simulink model "PIL_controller"  (R2022b)
settings: Solver=FixedStepAuto  StartTime=0.0  StopTime=10.0  FixedStep=0.01  RelTol=1e-3  EnableMultiTasking=on
libraries: pil_lib x1
settings Model: Creator=ok  LastModifiedBy=ok
settings OptimizationCC: EnhancedBackFolding=on  PassReuseOutputArgsAs=Individual arguments  ZeroExternalMemoryAtStartup=off  ZeroInternalMemoryAtStartup=off  MaxStackSize=64  OptimizeBlockOrder=speed  DifferentSizesBufferReuse=on  OptimizationCustomize=off  EfficientTunableParamExpr=on
settings DebuggingCC: ParameterTunabilityLossMsg=error
settings HardwareCC: ProdBitPerInt=16  ProdBitPerPointer=16  ProdBitPerSizeT=16  ProdBitPerPtrDiffT=16  ProdLargestAtomicFloat=None  ProdWordSize=8  ProdHWDeviceType=Atmel->AVR
settings SFSimCC: MATLABDynamicMemAlloc=off
settings RTWCC: Description=Embedded Coder  SystemTargetFile=ert.tlc  HardwareBoard=Arduino Uno  TLCOptions=-aInlineSetEventsForThisBaseRateFcn=TLC_FALSE -aSuppressMultiTaskScheduler=TLC_FALSE -aRateBasedStepFcn=1  TemplateMakefile=ert_default_tmf  Toolchain=Arduino AVR  BuildConfiguration=Faster Runs  CreateSILPILBlock=PIL
settings CodeAppCC: ForceParamTrailComments=on  IgnoreCustomStorageClasses=off  OperatorAnnotations=on  SimulinkDataObjDesc=on  SFDataObjDesc=on  InsertBlockDesc=on
settings ERTTargetCC: SupportContinuousTime=on  SupportVariableSizeSignals=on  ExtModeTransport=3  ExtModeStaticAlloc=on  ExtModeAutomaticAllocSize=off  ExtModeStaticAllocSize=250  ExtModeMexFile=ext_xcp  ExtModeIntrfLevel=Level2 - Open

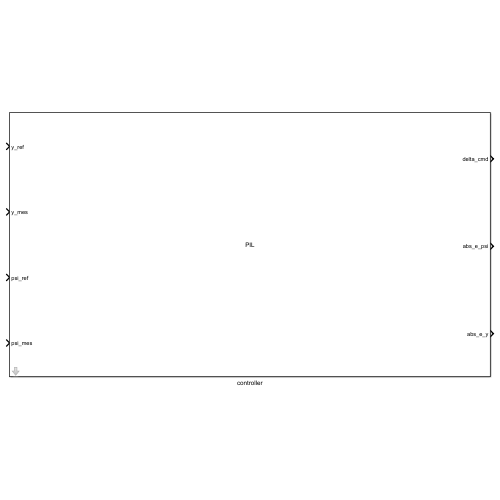
[thumbnail: Simulink's stored preview of the top-level diagram]
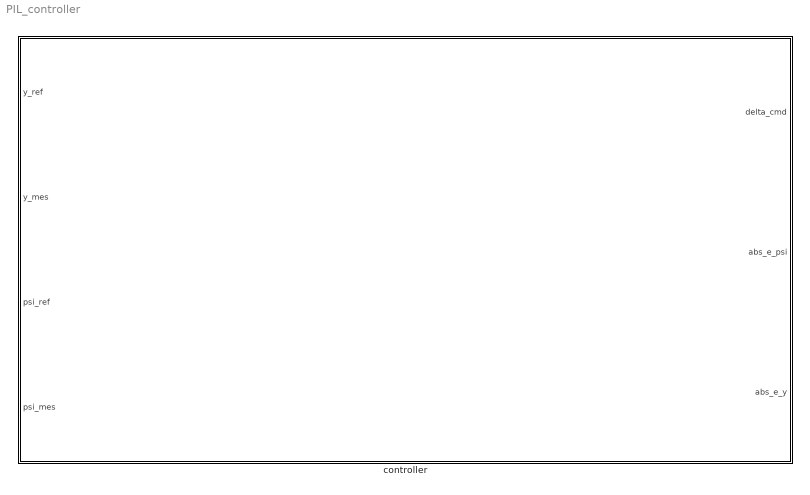
== system PIL_controller ==
  controller : Subsystem  DialogController=pil_create_dialog  LoadFcn=|
      | try
      |    if ~strcmp(rtw.pil.getPILVersion, '9.13 (R2022b)_15')
      |       set_param(gcb, 'DialogController', '');
      |       set_param(gcb, 'DialogControllerArgs', '');
      |    end
      | catch e
      |       set_param(gcb, 'DialogController', '');
      |       set_param(gcb, 'DialogControllerArgs', '');
      | end
      mask help: PIL:pil:XILBlockMaskDesc
      mask Display: disp('PIL');

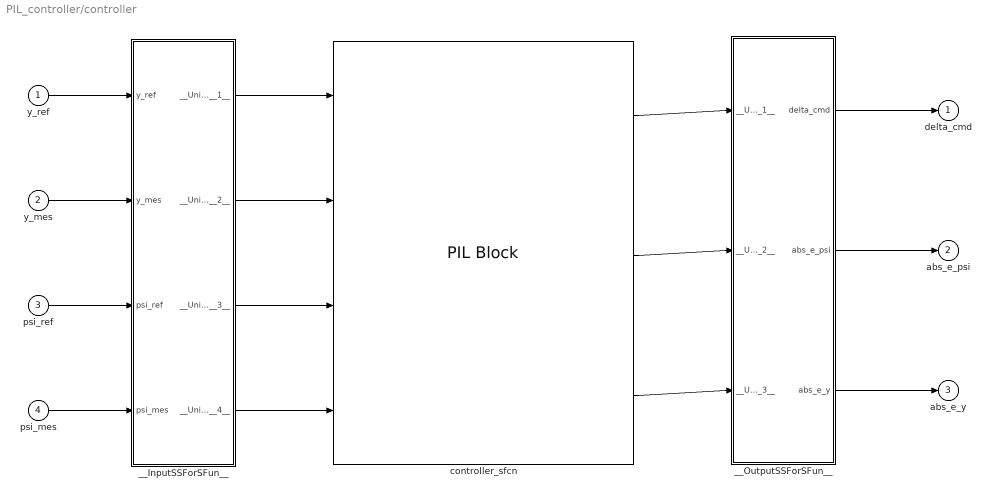
== system PIL_controller/controller ==
  y_ref : Inport
  y_mes : Inport  Port=2
  psi_ref : Inport  Port=3
  psi_mes : Inport  Port=4
  __InputSSForSFun__ : Subsystem
  __OutputSSForSFun__ : Subsystem
  controller_sfcn : pil_lib/PIL Block  SimulationMode=PIL  IsTopModelPIL=off  CodeDir=controller_ert_rtw  AnchorDir=C:\Users\ok\Documents\retest  ConfigName=Arduino Board  XrelIsTopModelCode=on  XrelIsReusable=off  XrelDWorkNames={}  XrelDWorkTypes={}  XrelModelArgVals={}  XrelOrderedParamNames={}
  delta_cmd : Outport
  abs_e_psi : Outport  Port=2
  abs_e_y : Outport  Port=3
  wires:
  y_ref/1 -> __InputSSForSFun__/1(y_ref)
  y_mes/1 -> __InputSSForSFun__/2(y_mes)
  psi_ref/1 -> __InputSSForSFun__/3(psi_ref)
  psi_mes/1 -> __InputSSForSFun__/4(psi_mes)
  __InputSSForSFun__/1(__UniqueOutportName__1__) -> controller_sfcn/1
  __InputSSForSFun__/2(__UniqueOutportName__2__) -> controller_sfcn/2
  __InputSSForSFun__/3(__UniqueOutportName__3__) -> controller_sfcn/3
  __InputSSForSFun__/4(__UniqueOutportName__4__) -> controller_sfcn/4
  controller_sfcn/1 -> __OutputSSForSFun__/1(__UniqueInportName__1__)
  controller_sfcn/2 -> __OutputSSForSFun__/2(__UniqueInportName__2__)
  controller_sfcn/3 -> __OutputSSForSFun__/3(__UniqueInportName__3__)
  __OutputSSForSFun__/1(delta_cmd) -> delta_cmd/1
  __OutputSSForSFun__/2(abs_e_psi) -> abs_e_psi/1
  __OutputSSForSFun__/3(abs_e_y) -> abs_e_y/1

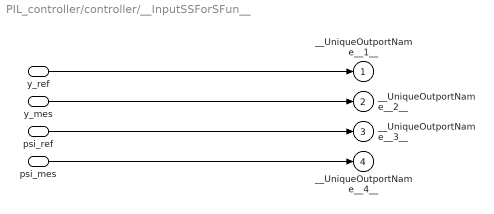
== system PIL_controller/controller/__InputSSForSFun__ ==
  y_ref : Inport
  y_mes : Inport  Port=2
  psi_ref : Inport  Port=3
  psi_mes : Inport  Port=4
  __UniqueOutportName__1__ : Outport
  __UniqueOutportName__2__ : Outport  Port=2
  __UniqueOutportName__3__ : Outport  Port=3
  __UniqueOutportName__4__ : Outport  Port=4
  wires:
  y_ref/1 -> __UniqueOutportName__1__/1
  y_mes/1 -> __UniqueOutportName__2__/1
  psi_ref/1 -> __UniqueOutportName__3__/1
  psi_mes/1 -> __UniqueOutportName__4__/1

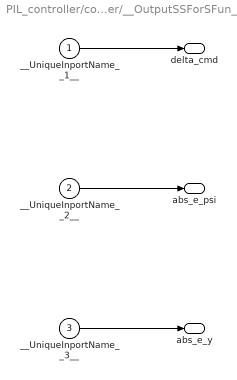
== system PIL_controller/controller/__OutputSSForSFun__ ==
  __UniqueInportName__1__ : Inport
  __UniqueInportName__2__ : Inport  Port=2
  __UniqueInportName__3__ : Inport  Port=3
  delta_cmd : Outport
  abs_e_psi : Outport  Port=2
  abs_e_y : Outport  Port=3
  wires:
  __UniqueInportName__1__/1 -> delta_cmd/1
  __UniqueInportName__2__/1 -> abs_e_psi/1
  __UniqueInportName__3__/1 -> abs_e_y/1
